simulink model "ball_and_plate_za_nn_2"  (R2018b)
settings: Solver=ode45  StartTime=0.0  StopTime=t_sim  RelTol=1e-3  EnableMultiTasking=on
values from neighbouring files (symbols this model uses):
  A_x = 0.05    [parametri.mat]    (also in proba_nn_simulink.m = 0.1; simulate_NOE_NARX_performance.mat = 0.1; simuliraj_kruznicu.m = radijus; test_nn_.m = 0.1)
  a_x = 0.388    [parametri.mat]    (also in simulate_NOE_NARX_performance.mat)
  A_y = 0.05    [parametri.mat]    (also in proba_nn_simulink.m = 0.1; simulate_NOE_NARX_performance.mat = 0.1; simuliraj_kruznicu.m = radijus; test_nn_.m = 0.1)
  a_y = 0.473    [parametri.mat]    (also in simulate_NOE_NARX_performance.mat)
  Ak_x = 0.1    [parametri.mat]    (also in simulate_NOE_NARX_performance.mat; simuliraj_kvadrat.m = stranica)
  Ak_y = 0.1    [parametri.mat]    (also in simulate_NOE_NARX_performance.mat; simuliraj_kvadrat.m = stranica)
  d = 2    [parametri.mat]    (also in simulate_NOE_NARX_performance.mat)
  Fc = 9.9675e-08    [parametri.mat]    (also in simulate_NOE_NARX_performance.mat)
  freq_x = 0.628318530718    [parametri.mat]    (also in simulate_NOE_NARX_performance.mat)
  freq_y = 0.628318530718    [parametri.mat]    (also in simulate_NOE_NARX_performance.mat)
  Fs = 1.9935e-07    [parametri.mat]    (also in simulate_NOE_NARX_performance.mat)
  g = 9.81    [parametri.mat]    (also in simulate_NOE_NARX_performance.mat)
  Jl = 7.48815837481e-05    [parametri.mat]    (also in simulate_NOE_NARX_performance.mat)
  konstanta = 0.1    [parametri.mat]    (also in simulate_NOE_NARX_performance.mat; simuliraj_kvadrat.m = 0.03)
  l = 0.1    [parametri.mat]    (also in simulate_NOE_NARX_performance.mat)
  ml = 0.0786597330257    [parametri.mat]    (also in simulate_NOE_NARX_performance.mat)
  odabir = 3    [proba_nn_simulink.m]    (also in simulate_NOE_NARX_performance.mat; simuliraj_kruznicu.m; simuliraj_kvadrat.m = 2; simuliraj_referenca.m = 1)
  period_x = 16    [parametri.mat]    (also in simulate_NOE_NARX_performance.mat)
  period_y = 16    [parametri.mat]    (also in simulate_NOE_NARX_performance.mat)
  phase_x = 1.57079632679    [parametri.mat]    (also in simulate_NOE_NARX_performance.mat)
  phase_y = 0    [parametri.mat]    (also in simulate_NOE_NARX_performance.mat)
  phasedelay_x = 0    [parametri.mat]    (also in simulate_NOE_NARX_performance.mat)
  phasedelay_y = 4    [parametri.mat]    (also in simulate_NOE_NARX_performance.mat)
  pw_x = 50    [parametri.mat]    (also in simulate_NOE_NARX_performance.mat)
  pw_y = 50    [parametri.mat]    (also in simulate_NOE_NARX_performance.mat)
  R = 0.0397    [parametri.mat]    (also in simulate_NOE_NARX_performance.mat)
  r = 0.02    [parametri.mat]    (also in simulate_NOE_NARX_performance.mat)
  t_step = 5    [parametri.mat]    (also in simulate_NOE_NARX_performance.mat)
  Td = 0.1    [parametri.mat]    (also in simulate_NOE_NARX_performance.mat)
  vs = 0.05    [parametri.mat]    (also in simulate_NOE_NARX_performance.mat)
  x0 = 0.15    [parametri.mat]    (also in proba_nn_simulink.m = a_x/2.0; simulate_NOE_NARX_performance.mat = 0.194; simuliraj_kruznicu.m = a_x/2.0; test_nn_.m = a_x/2.0)
  x0_loptica = 0.1    [proba_nn_simulink.m]    (also in simulate_NOE_NARX_performance.mat; simuliraj_kruznicu.m = x0_poc; simuliraj_kvadrat.m = x0_poc; simuliraj_referenca.m = x0_poc)
  x_step = 0.05    [parametri.mat]    (also in simulate_NOE_NARX_performance.mat; simuliraj_referenca.m = x_ref_value)
  y0 = 0.15    [parametri.mat]    (also in proba_nn_simulink.m = a_y/2.0; simulate_NOE_NARX_performance.mat = 0.2365; simuliraj_kruznicu.m = a_y/2.0; test_nn_.m = a_y/2.0)
  y0_loptica = 0.1    [proba_nn_simulink.m]    (also in simulate_NOE_NARX_performance.mat; simuliraj_kruznicu.m = y0_poc; simuliraj_kvadrat.m = y0_poc; simuliraj_referenca.m = y0_poc)
  y_step = 0.05    [parametri.mat]    (also in simulate_NOE_NARX_performance.mat; simuliraj_referenca.m = y_ref_value)
libraries: neural x118, simulink x6, fuzblock x2
(part 5 of 5)

== system ball_and_plate_za_nn_2/NOE/Layer 4/LW{4,3} ==
  "ad{4,3}" : Inport  PortDimensions=10  SampleTime=0.001
      mask Display: e = 0.06;c1 = [120 230 180]/255;c2 = ([120 230 180]+0)/(256+128);c3 = ([120 230 180]+128)/(256+128);patch([0 1 1 0],[0 0 1 1],c1);patch([0 1 1 1-e 1-e 0+e],[0 0 1 1-e 0+e 0+e],c2);patch([0 0 1 1-e 0+e 0+e],[0 1 1 1-e 1-e 0+e],c3);plot([0 1 1 0 0],[0 0 1 1 0]);
  "IW{4,3}(1,:)'" : Constant  Value=[0.40870539709809461381695427917293272912502288818359375;-0.2540888691627125606231629717512987554073333740234375;-0.57666466027429830187855941403540782630443572998046875;-0.80617111640670457983759433773229829967021942138671875;-0.3095025876504846618075816877535544335842132568359375;0.01232055950833396869292801767414857749827206134796142578125;0.91501847459988361332960948857362382113933563232421875;0.046476927022480130080595017716404981911182403564453125;-0.78709696630178560550206157131469808518886566162109375;0.2299334424622970496354668057392700575292110443115234375]
      mask Display: e = 0.06;c1 = [120 150 230]/255;c2 = ([120 150 230]+0)/383;c3 = ([120 150 230]+128)/383;patch([0 1 1 0],[0 0 1 1],c1);patch([0 1 1 1-e 1-e 0+e],[0 0 1 1-e 0+e 0+e],c2);patch([0 0 1 1-e 0+e 0+e],[0 1 1 1-e 1-e 0+e],c3);plot([0 1 1 0 0],[0 0 1 1 0]);disp('weights');
  "IW{4,3}(10,:)'" : Constant  Value=[0.391841205571248296646302833323716185986995697021484375;-0.77287431052964972177932168051484040915966033935546875;-0.2218660454561571515608164872901397757232189178466796875;-0.9501743690746662363011409979662857949733734130859375;-0.1314231945874096141313458474542130716145038604736328125;0.575969759172148432213589330785907804965972900390625;-0.50019731440796999510922660192591138184070587158203125;0.8354966701444543897281391764408908784389495849609375;-0.266684952879488401666918662158423103392124176025390625;0.60316473971497963635357564271544106304645538330078125]
      mask Display: e = 0.06;c1 = [120 150 230]/255;c2 = ([120 150 230]+0)/383;c3 = ([120 150 230]+128)/383;patch([0 1 1 0],[0 0 1 1],c1);patch([0 1 1 1-e 1-e 0+e],[0 0 1 1-e 0+e 0+e],c2);patch([0 0 1 1-e 0+e 0+e],[0 1 1 1-e 1-e 0+e],c3);plot([0 1 1 0 0],[0 0 1 1 0]);disp('weights');
  "IW{4,3}(2,:)'" : Constant  Value=[0.5417872549415123639704461311339400708675384521484375;0.26188639563861493275709335648571141064167022705078125;-1.060594195346266754853559177718125283718109130859375;-0.048002513012465684860696768510024412535130977630615234375;-0.1780902217946197796383245304241427220404148101806640625;0.054981556481401593072799727224264643155038356781005859375;-0.81666236417747395393007536767981946468353271484375;0.38904090476776287399474085759720765054225921630859375;-0.939386293784676862372862160555087029933929443359375;0.24049926258863651984398757122107781469821929931640625]
      mask Display: e = 0.06;c1 = [120 150 230]/255;c2 = ([120 150 230]+0)/383;c3 = ([120 150 230]+128)/383;patch([0 1 1 0],[0 0 1 1],c1);patch([0 1 1 1-e 1-e 0+e],[0 0 1 1-e 0+e 0+e],c2);patch([0 0 1 1-e 0+e 0+e],[0 1 1 1-e 1-e 0+e],c3);plot([0 1 1 0 0],[0 0 1 1 0]);disp('weights');
  "IW{4,3}(3,:)'" : Constant  Value=[0.000939344033684942798789752060883984086103737354278564453125;0.84524127369610091431439968800987116992473602294921875;-0.3941174691466595714217646673205308616161346435546875;1.0034068425839268723365194091456942260265350341796875;0.231753049913562048089943345985375344753265380859375;-0.5192550117031713430293393685133196413516998291015625;-0.208887211309706610773417878590407781302928924560546875;0.28539820305701379954399499183637090027332305908203125;0.77759269305989831000403000871301628649234771728515625;0.381779872290980482052447086971369571983814239501953125]
      mask Display: e = 0.06;c1 = [120 150 230]/255;c2 = ([120 150 230]+0)/383;c3 = ([120 150 230]+128)/383;patch([0 1 1 0],[0 0 1 1],c1);patch([0 1 1 1-e 1-e 0+e],[0 0 1 1-e 0+e 0+e],c2);patch([0 0 1 1-e 0+e 0+e],[0 1 1 1-e 1-e 0+e],c3);plot([0 1 1 0 0],[0 0 1 1 0]);disp('weights');
  "IW{4,3}(4,:)'" : Constant  Value=[-0.06791209967671564540214745875346125103533267974853515625;0.66430400356172680798039209548733197152614593505859375;-0.25316358100225777594260989644681103527545928955078125;-0.351702647292925385524853254537447355687618255615234375;0.87479107515515075466083771971170790493488311767578125;-0.94018974009686306914090891950763761997222900390625;0.795091425512663096952792329830117523670196533203125;0.210380897711272163430606951806112192571163177490234375;-0.5296542738384466542100881270016543567180633544921875;0.2220539022214716162739733817943488247692584991455078125]
      mask Display: e = 0.06;c1 = [120 150 230]/255;c2 = ([120 150 230]+0)/383;c3 = ([120 150 230]+128)/383;patch([0 1 1 0],[0 0 1 1],c1);patch([0 1 1 1-e 1-e 0+e],[0 0 1 1-e 0+e 0+e],c2);patch([0 0 1 1-e 0+e 0+e],[0 1 1 1-e 1-e 0+e],c3);plot([0 1 1 0 0],[0 0 1 1 0]);disp('weights');
  "IW{4,3}(5,:)'" : Constant  Value=[0.1767258987712781170831277677280013449490070343017578125;0.91630858276520676941601095677469857037067413330078125;0.2007543073089513574469577861236757598817348480224609375;0.154980445589328663658079676679335534572601318359375;-0.1683306701251934267560272928676567971706390380859375;-0.84826572881355699617955679059377871453762054443359375;0.293111189214277256809282334870658814907073974609375;-0.20264528265917858274036689181230030953884124755859375;-1.01057004139361961136955869733355939388275146484375;-0.08291356458034003507062692506224266253411769866943359375]
      mask Display: e = 0.06;c1 = [120 150 230]/255;c2 = ([120 150 230]+0)/383;c3 = ([120 150 230]+128)/383;patch([0 1 1 0],[0 0 1 1],c1);patch([0 1 1 1-e 1-e 0+e],[0 0 1 1-e 0+e 0+e],c2);patch([0 0 1 1-e 0+e 0+e],[0 1 1 1-e 1-e 0+e],c3);plot([0 1 1 0 0],[0 0 1 1 0]);disp('weights');
  "IW{4,3}(6,:)'" : Constant  Value=[0.54328328957335891846724962306325323879718780517578125;0.691608251953872876782725143129937350749969482421875;0.6078641552083838828224315875559113919734954833984375;0.25679773545168027570895219469093717634677886962890625;-0.054190034319975328991336738226891611702740192413330078125;0.6238359561945963083218202882562763988971710205078125;0.81508785066547806419379185172147117555141448974609375;-0.453777327654840856308027241539093665778636932373046875;0.56547815556141733939199411906884051859378814697265625;-0.5938651505074663550232116904226131737232208251953125]
      mask Display: e = 0.06;c1 = [120 150 230]/255;c2 = ([120 150 230]+0)/383;c3 = ([120 150 230]+128)/383;patch([0 1 1 0],[0 0 1 1],c1);patch([0 1 1 1-e 1-e 0+e],[0 0 1 1-e 0+e 0+e],c2);patch([0 0 1 1-e 0+e 0+e],[0 1 1 1-e 1-e 0+e],c3);plot([0 1 1 0 0],[0 0 1 1 0]);disp('weights');
  "IW{4,3}(7,:)'" : Constant  Value=[0.416922666869295743818923938306397758424282073974609375;0.79366518187884260715492246163194067776203155517578125;-0.484883128064957535929835330534842796623706817626953125;-0.1164025271941328265601356406477862037718296051025390625;0.6113968684917006068957334719016216695308685302734375;-0.66721431902438299577084990232833661139011383056640625;-0.044172263035992830049192292563020600937306880950927734375;-0.1867029155844549814791122344104223884642124176025390625;-0.88087186787475157956350813037715852260589599609375;0.63456291886210280939195627070148475468158721923828125]
      mask Display: e = 0.06;c1 = [120 150 230]/255;c2 = ([120 150 230]+0)/383;c3 = ([120 150 230]+128)/383;patch([0 1 1 0],[0 0 1 1],c1);patch([0 1 1 1-e 1-e 0+e],[0 0 1 1-e 0+e 0+e],c2);patch([0 0 1 1-e 0+e 0+e],[0 1 1 1-e 1-e 0+e],c3);plot([0 1 1 0 0],[0 0 1 1 0]);disp('weights');
  "IW{4,3}(8,:)'" : Constant  Value=[0.044487985093605221520451920014238567091524600982666015625;-0.8464129571423535391971881836070679128170013427734375;-0.10913072854795903554592229056652286089956760406494140625;-0.1547982046578038894946161008192575536668300628662109375;-0.1417084793712377333019247771517257206141948699951171875;0.5689093401124012405745133946766145527362823486328125;-0.85969885445430749282280658007948659360408782958984375;-0.8234758079399835395406626048497855663299560546875;0.64619184530852680214962902027764357626438140869140625;-0.445754039863237749852231672775815241038799285888671875]
      mask Display: e = 0.06;c1 = [120 150 230]/255;c2 = ([120 150 230]+0)/383;c3 = ([120 150 230]+128)/383;patch([0 1 1 0],[0 0 1 1],c1);patch([0 1 1 1-e 1-e 0+e],[0 0 1 1-e 0+e 0+e],c2);patch([0 0 1 1-e 0+e 0+e],[0 1 1 1-e 1-e 0+e],c3);plot([0 1 1 0 0],[0 0 1 1 0]);disp('weights');
  "IW{4,3}(9,:)'" : Constant  Value=[-0.36253332852955555409835142199881374835968017578125;-0.86417254264218901216310086965677328407764434814453125;0.61938491178412935500574576508370228111743927001953125;0.79094265482623649088367301374091766774654388427734375;0.63959137502408525133290595476864837110042572021484375;0.382269537268440540156433371521416120231151580810546875;0.2201585580218360649329412126462557353079319000244140625;0.1824392069742414579369693683474906720221042633056640625;-0.70387644815780425755491478412295691668987274169921875;0.27393026557719812874580611605779267847537994384765625]
      mask Display: e = 0.06;c1 = [120 150 230]/255;c2 = ([120 150 230]+0)/383;c3 = ([120 150 230]+128)/383;patch([0 1 1 0],[0 0 1 1],c1);patch([0 1 1 1-e 1-e 0+e],[0 0 1 1-e 0+e 0+e],c2);patch([0 0 1 1-e 0+e 0+e],[0 1 1 1-e 1-e 0+e],c3);plot([0 1 1 0 0],[0 0 1 1 0]);disp('weights');
  Mux : Mux  Inputs=10
      mask Display: e = 0.06;c1 = [120 150 230]/255;c2 = ([120 150 230]+0)/383;c3 = ([120 150 230]+128)/383;patch([0 1 1 0],[0 0 1 1],c1);patch([0 1 1 1-e 1-e 0+e],[0 0 1 1-e 0+e 0+e],c2);patch([0 0 1 1-e 0+e 0+e],[0 1 1 1-e 1-e 0+e],c3);plot([0 1 1 0 0],[0 0 1 1 0]);disp('Mux');
  dotprod{1..10} (10 alike) : neural/Weight Functions/dotprod
  "lz{4,3}" : Outport
      mask Display: e = 0.06;c1 = [120 230 180]/255;c2 = ([120 230 180]+0)/(256+128);c3 = ([120 230 180]+128)/(256+128);patch([0 1 1 0],[0 0 1 1],c1);patch([0 1 1 1-e 1-e 0+e],[0 0 1 1-e 0+e 0+e],c2);patch([0 0 1 1-e 0+e 0+e],[0 1 1 1-e 1-e 0+e],c3);plot([0 1 1 0 0],[0 0 1 1 0]);
  wires:
  "IW{4,3}(1,:)'"/1 -> dotprod1/1
  "ad{4,3}"/1 -> dotprod1/2, dotprod2/2, dotprod3/2, dotprod4/2, dotprod5/2, dotprod6/2, dotprod7/2, dotprod8/2, dotprod9/2, dotprod10/2
  dotprod1/1 -> Mux/1
  "IW{4,3}(2,:)'"/1 -> dotprod2/1
  dotprod2/1 -> Mux/2
  "IW{4,3}(3,:)'"/1 -> dotprod3/1
  dotprod3/1 -> Mux/3
  "IW{4,3}(4,:)'"/1 -> dotprod4/1
  dotprod4/1 -> Mux/4
  "IW{4,3}(5,:)'"/1 -> dotprod5/1
  dotprod5/1 -> Mux/5
  "IW{4,3}(6,:)'"/1 -> dotprod6/1
  dotprod6/1 -> Mux/6
  "IW{4,3}(7,:)'"/1 -> dotprod7/1
  dotprod7/1 -> Mux/7
  "IW{4,3}(8,:)'"/1 -> dotprod8/1
  dotprod8/1 -> Mux/8
  "IW{4,3}(9,:)'"/1 -> dotprod9/1
  dotprod9/1 -> Mux/9
  "IW{4,3}(10,:)'"/1 -> dotprod10/1
  dotprod10/1 -> Mux/10
  Mux/1 -> "lz{4,3}"/1

== system ball_and_plate_za_nn_2/NOE/Layer 5/Delays 1 ==
  "p{5}" : Inport  PortDimensions=10  SampleTime=0.001
      mask Display: e = 0.06;c1 = [120 230 180]/255;c2 = ([120 230 180]+0)/(256+128);c3 = ([120 230 180]+128)/(256+128);patch([0 1 1 0],[0 0 1 1],c1);patch([0 1 1 1-e 1-e 0+e],[0 0 1 1-e 0+e 0+e],c2);patch([0 0 1 1-e 0+e 0+e],[0 1 1 1-e 1-e 0+e],c3);plot([0 1 1 0 0],[0 0 1 1 0]);
  mux : Mux  Inputs=1
      mask Display: e = 0.06;c1 = [120 150 230]/255;c2 = ([120 150 230]+0)/383;c3 = ([120 150 230]+128)/383;patch([0 1 1 0],[0 0 1 1],c1);patch([0 1 1 1-e 1-e 0+e],[0 0 1 1-e 0+e 0+e],c2);patch([0 0 1 1-e 0+e 0+e],[0 1 1 1-e 1-e 0+e],c3);plot([0 1 1 0 0],[0 0 1 1 0]);disp('Mux')
  "pd{5,4}" : Outport
      mask Display: e = 0.06;c1 = [120 230 180]/255;c2 = ([120 230 180]+0)/(256+128);c3 = ([120 230 180]+128)/(256+128);patch([0 1 1 0],[0 0 1 1],c1);patch([0 1 1 1-e 1-e 0+e],[0 0 1 1-e 0+e 0+e],c2);patch([0 0 1 1-e 0+e 0+e],[0 1 1 1-e 1-e 0+e],c3);plot([0 1 1 0 0],[0 0 1 1 0]);
  wires:
  "p{5}"/1 -> mux/1
  mux/1 -> "pd{5,4}"/1

== system ball_and_plate_za_nn_2/NOE/Layer 5/LW{5,4} ==
  "ad{5,4}" : Inport  PortDimensions=10  SampleTime=0.001
      mask Display: e = 0.06;c1 = [120 230 180]/255;c2 = ([120 230 180]+0)/(256+128);c3 = ([120 230 180]+128)/(256+128);patch([0 1 1 0],[0 0 1 1],c1);patch([0 1 1 1-e 1-e 0+e],[0 0 1 1-e 0+e 0+e],c2);patch([0 0 1 1-e 0+e 0+e],[0 1 1 1-e 1-e 0+e],c3);plot([0 1 1 0 0],[0 0 1 1 0]);
  "IW{5,4}(1,:)'" : Constant  Value=[-0.5993186560139383001200030776089988648891448974609375;1.15220156548277685715220286510884761810302734375;-1.04801006435799326510505125042982399463653564453125;0.588818598760254108270828510285355150699615478515625;0.81314572435573106989892266938113607466220855712890625;-0.90504484675990093389685853253467939794063568115234375;0.0700781095534457609819156687080976553261280059814453125;0.7012762669828094264090623255469836294651031494140625;-0.207290568772410421782836920101544819772243499755859375;0.62453079569397573767020048762788064777851104736328125]
      mask Display: e = 0.06;c1 = [120 150 230]/255;c2 = ([120 150 230]+0)/383;c3 = ([120 150 230]+128)/383;patch([0 1 1 0],[0 0 1 1],c1);patch([0 1 1 1-e 1-e 0+e],[0 0 1 1-e 0+e 0+e],c2);patch([0 0 1 1-e 0+e 0+e],[0 1 1 1-e 1-e 0+e],c3);plot([0 1 1 0 0],[0 0 1 1 0]);disp('weights');
  Mux : Mux  Inputs=1
      mask Display: e = 0.06;c1 = [120 150 230]/255;c2 = ([120 150 230]+0)/383;c3 = ([120 150 230]+128)/383;patch([0 1 1 0],[0 0 1 1],c1);patch([0 1 1 1-e 1-e 0+e],[0 0 1 1-e 0+e 0+e],c2);patch([0 0 1 1-e 0+e 0+e],[0 1 1 1-e 1-e 0+e],c3);plot([0 1 1 0 0],[0 0 1 1 0]);disp('Mux');
  dotprod1 : neural/Weight Functions/dotprod
  "lz{5,4}" : Outport
      mask Display: e = 0.06;c1 = [120 230 180]/255;c2 = ([120 230 180]+0)/(256+128);c3 = ([120 230 180]+128)/(256+128);patch([0 1 1 0],[0 0 1 1],c1);patch([0 1 1 1-e 1-e 0+e],[0 0 1 1-e 0+e 0+e],c2);patch([0 0 1 1-e 0+e 0+e],[0 1 1 1-e 1-e 0+e],c3);plot([0 1 1 0 0],[0 0 1 1 0]);
  wires:
  "IW{5,4}(1,:)'"/1 -> dotprod1/1
  "ad{5,4}"/1 -> dotprod1/2
  dotprod1/1 -> Mux/1
  Mux/1 -> "lz{5,4}"/1
